simulink model "attitude_controller"  (R2012b)
settings: Solver=FixedStepDiscrete  SolverMode=SingleTasking  StartTime=0.0  StopTime=25  FixedStep=1/40  RelTol=1e-3
model workspace (MAT data in the model file):
  dispGain = Simulink.Parameter
  dispGain.Value = 0.75
  dispGain.Description = 'This is the gain applied to the displacement error.'
  dispGain.DataType = 'auto'
  dispGain.Min = 0
  dispGain.DocUnits = 'deg/sec/deg'
  dispLim = Simulink.Parameter
  dispLim.Value = 30
  dispLim.Description = 'This is the limit for controlling the maximum commanded angle.'
  dispLim.DataType = 'auto'
  dispLim.Min = 0
  dispLim.Max = 180
  dispLim.DocUnits = 'deg'
  rateGain = Simulink.Parameter
  rateGain.Value = 2
  rateGain.Description = 'This is the gain applied to the rate error.'
  rateGain.DataType = 'auto'
  rateGain.Min = 0
  rateGain.DocUnits = 'deg/deg/sec'
  rateLim = Simulink.Parameter
  rateLim.Value = 6
  rateLim.Description = 'This is the limit for controlling the maximum commanded angle.'
  rateLim.DataType = 'auto'
  rateLim.Min = 0
  rateLim.Max = 180
  rateLim.DocUnits = 'deg/sec'
  intGain = Simulink.Parameter
  intGain.Value = 0.5
  intGain.Description = 'This is the gain applied to the integral error.'
  intGain.DataType = 'auto'
  intGain.Min = 0
  intGain.DocUnits = 'deg/sec/deg/sec'
  intLim = Simulink.Parameter
  intLim.Value = 5
  intLim.Description = 'This is the limit for controlling the maximum commanded angle.'
  intLim.DataType = 'auto'
  intLim.Min = 0
  intLim.Max = 90
  intLim.DocUnits = 'deg'
  cmdLim = Simulink.Parameter
  cmdLim.Value = 15
  cmdLim.Description = 'This is the limit for controlling the maximum surface command angle.'
  cmdLim.DataType = 'auto'
  cmdLim.Min = 0
  cmdLim.Max = 90
  cmdLim.DocUnits = 'deg'
undefined symbols (not defined in the file or in its folder): DiscIntNeverNeededParam
libraries: simulink x1
settings Model: RequirementInfo={'doors' '00000040' '1' 'false' 'DOORS Surrogate Item' '' } %GIDa_eb906a4c_0ec7_43a1_b5c3_86a9990349a4  FPTRunName=FPA_Reference  reqMgrSettings="100 S'doors','misc'{{S'surrogatepath','savemodel','savesurrogate','doorsLinks2sl','slLinks2Doors','detaillevel','surrogateId','synctime'{{T\"/Autopilot Project/attitude_controller\",M[1],M[1],M[1],M[1],M[1],T\"00000040\",T\"\"}},S'mode','pathStorage'{{T\"generic\",T\"modelRelative\"}}}}"  CovSaveName=attitude_controller_covdata  CovMetricSettings=dcmtrwe  CovHTMLOptions=-aTS=1 -bRG=1 -bTC=1 -hTR=1 -nFC=0 -scm=1 -bcm=1  CovHtmlReporting=off  CovCumulativeVarName=attitude_controller_covCumulativeData  CovCumulativeReport=on  CovReportOnPause=off  CovModelRefEnable=off  Creator=bpotter  LastModifiedBy=bpotter
settings DataIOCC: ExternalInput=attitudeIn  LimitDataPoints=off  SaveFormat=StructureWithTime  SignalLoggingSaveFormat=ModelDataLogs  SaveOutput=off  SignalLogging=off  SaveTime=off
settings OptimizationCC: BlockReduction=off  InlineParams=on  InlineInvariantSignals=on  EfficientFloat2IntCast=on  EfficientMapNaN2IntZero=off  OptimizeModelRefInitCode=on  MaxStackSize=inf
settings DebuggingCC: SignalInfNanChecking=error  SignalRangeChecking=error  ReadBeforeWriteMsg=EnableAllAsError  WriteAfterWriteMsg=EnableAllAsError  WriteAfterReadMsg=EnableAllAsError  AlgebraicLoopMsg=error  ArtificialAlgebraicLoopMsg=error  SaveWithDisabledLinksMsg=error  SaveWithParameterizedLinksMsg=error  UnderspecifiedInitializationDetection=Simplified  CheckExecutionContextPreStartOutputMsg=on  CheckExecutionContextRuntimeOutputMsg=on  BlockPriorityViolationMsg=error  MaxConsecutiveZCsMsg=warning  SolverPrmCheckMsg=error  InheritedTsInSrcMsg=error  DiscreteInheritContinuousMsg=error  SingleTaskRateTransMsg=error  TasksWithSamePriorityMsg=error  SigSpecEnsureSampleTimeMsg=error  CheckMatrixSingularityMsg=error  IntegerOverflowMsg=error  ParameterUnderflowMsg=error  ParameterPrecisionLossMsg=error  ParameterTunabilityLossMsg=error  UnderSpecifiedDataTypeMsg=error  UnnecessaryDatatypeConvMsg=warning  VectorMatrixConversionMsg=error  SignalLabelMismatchMsg=error  UnconnectedInputMsg=error  UnconnectedOutputMsg=error  UnconnectedLineMsg=error  SFcnCompatibilityMsg=error  UniqueDataStoreMsg=error  BusObjectLabelMismatch=error  RootOutportRequireBusObject=error  AssertControl=DisableAll  ModelReferenceIOMsg=error  ModelReferenceIOMismatchMessage=error  ModelReferenceCSMismatchMessage=warning  UnknownTsInhSupMsg=error  ModelReferenceDataLoggingMessage=error  ModelReferenceExtraNoncontSigs=none  StrictBusMsg=ErrorOnBusTreatedAsVector  NonBusSignalsTreatedAsBus=error
settings HardwareCC: ProdIntDivRoundTo=Zero  ProdEndianess=BigEndian  ProdHWDeviceType=32-bit Embedded Processor  TargetHWDeviceType=32-bit Generic
settings RTWCC: SystemTargetFile=ert.tlc  GenCodeOnly=on  GenerateMakefile=off  TemplateMakefile=ert_default_tmf  Description=Embedded Coder  GenerateReport=on  RTWVerbose=off  ProcessScript=ert_make_rtw_hook  IncludeHyperlinkInReport=on  LaunchReport=on  GenerateTraceInfo=on  GenerateTraceReport=on  GenerateTraceReportSl=on  GenerateTraceReportSf=on  GenerateTraceReportEml=on
settings CodeAppCC: ForceParamTrailComments=on  IgnoreCustomStorageClasses=off  MaxIdLength=63  MangleLength=4  ReqsInCode=on
settings ERTTargetCC: CodeReplacementLibrary=ANSI_C  UtilityFuncGeneration=Shared location  MultiwordLength=2048  IncludeMdlTerminateFcn=off  GeneratePreprocessorConditionals=Disable all  SuppressErrorStatus=on  SupportAbsoluteTime=off  MultiInstanceERTCode=on  SupportNonFinite=off  SupportComplex=off  ParenthesesLevel=Maximum  InlinedParameterPlacement=NonHierarchical  MultiInstanceErrorCode=None  ERTCustomFileTemplate=example_file_process.tlc  PreserveExpressionOrder=on  PreserveIfCondition=on  ConvertIfToSwitch=off  SuppressUnreachableDefaultCases=off

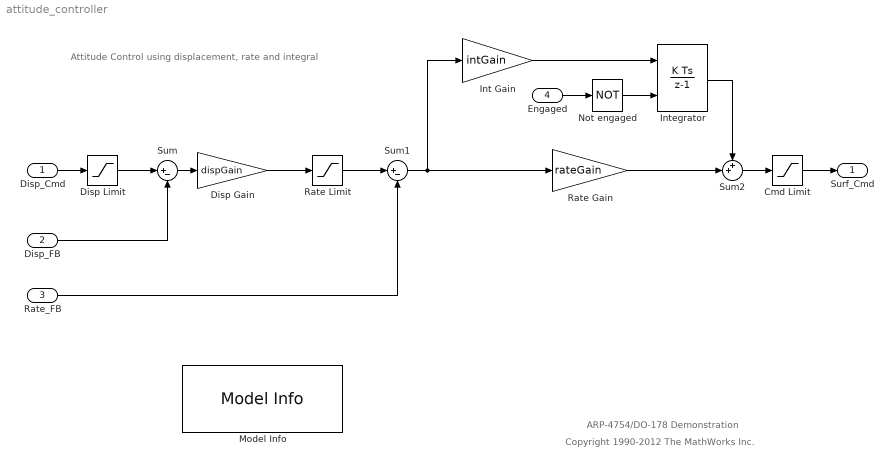
== system attitude_controller ==
  note: Attitude Control using displacement, rate and integral
  note: Copyright 1990-2012 The MathWorks Inc.
  note: ARP-4754/DO-178 Demonstration
  Disp_Cmd : Inport  RequirementInfo={'doors' '00000040' '2' 'false' '1.1 Disp_Cmd' '' ; 'linktype_rmi_doors' '00000020 (/Autopilot/Attitude Controller Derived Requirements)' '#22' 'true' '2.1.1 Inputs' '' } %GIDa_1f6c7271_93c3_4f3b_ad46_40b2620097e5  OutDataTypeStr=double  PortDimensions=1  SampleTime=1/40
  "Disp_FB " : Inport  RequirementInfo={'doors' '00000040' '3' 'false' '1.2 Disp_FB ' '' ; 'linktype_rmi_doors' '00000020 (/Autopilot/Attitude Controller Derived Requirements)' '#22' 'true' '2.1.1 Inputs' '' } %GIDa_a4c10b54_79b2_494f_9fbb_11aba459525d  Port=2  OutDataTypeStr=double  PortDimensions=1  SampleTime=1/40
  Rate_FB : Inport  RequirementInfo={'doors' '00000040' '4' 'false' '1.3 Rate_FB' '' ; 'linktype_rmi_doors' '00000020 (/Autopilot/Attitude Controller Derived Requirements)' '#22' 'true' '2.1.1 Inputs' '' } %GIDa_8a5ee350_5b96_4034_aa7b_307fc7a5da71  Port=3  OutDataTypeStr=double  PortDimensions=1  SampleTime=1/40
  Engaged : Inport  RequirementInfo={'doors' '00000040' '5' 'false' '1.4 Engaged' '' ; 'linktype_rmi_doors' '00000020 (/Autopilot/Attitude Controller Derived Requirements)' '#22' 'true' '2.1.1 Inputs' '' } %GIDa_99509e30_ac8c_4d41_82c3_48695d972b31  Port=4  OutDataTypeStr=boolean  PortDimensions=1  SampleTime=1/40
  Cmd Limit : Saturate  RequirementInfo={'doors' '00000040' '6' 'false' '1.5 Cmd Limit' '' ; 'linktype_rmi_doors' '00000020 (/Autopilot/Attitude Controller Derived Requirements)' '#23' 'true' '2.1.2 Parameters' '' ; 'linktype_rmi_doors' '00000020 (/Autopilot/Attitude Controller Derived Requirements)' '#21' 'true' '2.5 Surface Command and Limit' '' } %GIDa_ec5fb8d1_63e1_4cbf_bd50_e97ea1f3a86f  UpperLimit=cmdLim  LowerLimit=-cmdLim
      settings: AttributesFormatString=%<LowerLimit> to %<UpperLimit> (deg)
  Disp Gain : Gain  RequirementInfo={'doors' '00000040' '7' 'false' '1.6 Disp Gain' '' ; 'linktype_rmi_doors' '00000020 (/Autopilot/Attitude Controller Derived Requirements)' '#23' 'true' '2.1.2 Parameters' '' ; 'linktype_rmi_doors' '00000020 (/Autopilot/Attitude Controller Derived Requirements)' '#16' 'true' '2.2 Attitude Control and Limit' '' } %GIDa_4fcfcfe9_3275_4fa9_885f_cf306a71b936  Gain=dispGain
  Disp Limit : Saturate  RequirementInfo={'doors' '00000040' '8' 'false' '1.7 Disp Limit' '' ; 'linktype_rmi_doors' '00000020 (/Autopilot/Attitude Controller Derived Requirements)' '#23' 'true' '2.1.2 Parameters' '' ; 'linktype_rmi_doors' '00000020 (/Autopilot/Attitude Controller Derived Requirements)' '#16' 'true' '2.2 Attitude Control and Limit' '' } %GIDa_7b92da27_c5ec_485b_a9fa_f73a890a94ea  UpperLimit=dispLim  LowerLimit=-dispLim
      settings: AttributesFormatString=%<LowerLimit> to %<UpperLimit> (deg)
  Int Gain : Gain  RequirementInfo={'doors' '00000040' '9' 'false' '1.8 Int Gain' '' ; 'linktype_rmi_doors' '00000020 (/Autopilot/Attitude Controller Derived Requirements)' '#23' 'true' '2.1.2 Parameters' '' ; 'linktype_rmi_doors' '00000020 (/Autopilot/Attitude Controller Derived Requirements)' '#20' 'true' '2.4 Integral Control and Limit' '' } %GIDa_beea6fba_2894_42ca_8163_07bc86b02f8e  Gain=intGain
  Integrator : DiscreteIntegrator  RequirementInfo={'doors' '00000040' '10' 'false' '1.9 Integrator' '' ; 'linktype_rmi_doors' '00000020 (/Autopilot/Attitude Controller Derived Requirements)' '#23' 'true' '2.1.2 Parameters' '' ; 'linktype_rmi_doors' '00000020 (/Autopilot/Attitude Controller Derived Requirements)' '#20' 'true' '2.4 Integral Control and Limit' '' } %GIDa_56920583_9fba_490e_bbc1_cc2be4dd2810  ExternalReset=level  SampleTime=1/40  LimitOutput=on  UpperSaturationLimit=intLim  LowerSaturationLimit=-intLim  IgnoreLimit=on  ICPrevOutput=DiscIntNeverNeededParam  ICPrevScaledInput=DiscIntNeverNeededParam
      settings: AttributesFormatString=%<LowerSaturationLimit> to %<UpperSaturationLimit> (deg)
  Model Info : simulink/Model-Wide Utilities/Model Info  InitialBlockCM=None  BlockCM=None  Frame=on  DisplayStringWithTags=|  HorizontalTextAlignment=Left  LeftAlignmentValue=0.02  SourceBlockDiagram=attitude_controller  TagMaxNumber=20
      | Attitude Controller
      | Author: %<LastModifiedBy>
      | Version: %<ModelVersion>
      | Date: %<LastModificationDate>
  Not engaged : Logic  RequirementInfo={'doors' '00000040' '11' 'false' '1.10 Not engaged' '' ; 'linktype_rmi_doors' '00000020 (/Autopilot/Attitude Controller Derived Requirements)' '#20' 'true' '2.4 Integral Control and Limit' '' } %GIDa_955db51c_db14_42aa_b67d_de05482530f8  Operator=NOT  IconShape=distinctive  AllPortsSameDT=off  OutDataTypeStr=boolean
  Rate Gain : Gain  RequirementInfo={'doors' '00000040' '12' 'false' '1.11 Rate Gain' '' ; 'linktype_rmi_doors' '00000020 (/Autopilot/Attitude Controller Derived Requirements)' '#23' 'true' '2.1.2 Parameters' '' ; 'linktype_rmi_doors' '00000020 (/Autopilot/Attitude Controller Derived Requirements)' '#18' 'true' '2.3 Rate Control and Limit' '' } %GIDa_4fe20f02_adbd_4ca0_a7f6_fed161d48486  Gain=rateGain
  Rate Limit : Saturate  RequirementInfo={'doors' '00000040' '13' 'false' '1.12 Rate Limit' '' ; 'linktype_rmi_doors' '00000020 (/Autopilot/Attitude Controller Derived Requirements)' '#23' 'true' '2.1.2 Parameters' '' ; 'linktype_rmi_doors' '00000020 (/Autopilot/Attitude Controller Derived Requirements)' '#18' 'true' '2.3 Rate Control and Limit' '' } %GIDa_6ae337a4_f989_4d2e_9517_e05a98139e9b  UpperLimit=rateLim  LowerLimit=-rateLim
      settings: AttributesFormatString=%<LowerLimit> to %<UpperLimit> (deg/sec)
  Sum : Sum  RequirementInfo={'doors' '00000040' '14' 'false' '1.13 Sum' '' ; 'linktype_rmi_doors' '00000020 (/Autopilot/Attitude Controller Derived Requirements)' '#16' 'true' '2.2 Attitude Control and Limit' '' } %GIDa_cf5e480a_5b22_4e1a_9467_aeba7515f114  Inputs=|+-
  Sum1 : Sum  RequirementInfo={'doors' '00000040' '15' 'false' '1.14 Sum1' '' ; 'linktype_rmi_doors' '00000020 (/Autopilot/Attitude Controller Derived Requirements)' '#18' 'true' '2.3 Rate Control and Limit' '' } %GIDa_37a43aee_ff03_4021_a10a_39656d6638a3  Inputs=|+-
  Sum2 : Sum  RequirementInfo={'doors' '00000040' '16' 'false' '1.15 Sum2' '' ; 'linktype_rmi_doors' '00000020 (/Autopilot/Attitude Controller Derived Requirements)' '#21' 'true' '2.5 Surface Command and Limit' '' } %GIDa_fadb0a26_a1fd_480b_9f5d_0b7f45001c5e  Inputs=++|
  Surf_Cmd : Outport  RequirementInfo={'doors' '00000040' '17' 'false' '1.16 Surf_Cmd' '' ; 'linktype_rmi_doors' '00000020 (/Autopilot/Attitude Controller Derived Requirements)' '#24' 'true' '2.1.3 Outputs' '' } %GIDa_99d2b8ce_ab27_4685_9887_a082a0698432  OutDataTypeStr=double  PortDimensions=1  SampleTime=1/40
  wires:
  Disp_Cmd/1 -> Disp Limit/1
  "Disp_FB "/1 -> Sum/2
  Rate_FB/1 -> Sum1/2
  Sum1/1 -> Rate Gain/1, Int Gain/1
  Disp Gain/1 -> Rate Limit/1
  Sum/1 -> Disp Gain/1
  Disp Limit/1 -> Sum/1
  Rate Limit/1 -> Sum1/1
  Cmd Limit/1 -> Surf_Cmd/1
  Rate Gain/1 -> Sum2/2
  Sum2/1 -> Cmd Limit/1
  Engaged/1 -> Not engaged/1
  Not engaged/1 -> Integrator/2
  Integrator/1 -> Sum2/1
  Int Gain/1 -> Integrator/1
